simulink model "SerialMaster"  (R2023b)
settings: Solver=FixedStepAuto  StartTime=0.0  StopTime=10.0  FixedStep=1e-3  RelTol=1e-3  EnableMultiTasking=on
undefined symbols (not defined in the file or in its folder): D0, D1, D10, D11, D12, D13, D2, D3, D4, D5, D6, D7, D8, D9, PTA0, PTA1, PTA2, PTB23, PTB9, PTC16, PTC17, PTC2, PTC3, PTC4, PTD0, PTD1, PTD2, PTD3
libraries: frdmk64flib x20, etargetslib x9, dspstat3 x1
settings Model: ExtModeTrigDuration=5  Creator=Mathew  LastModifiedBy=Mathew
settings DataIOCC: InspectSignalLogs=on
settings OptimizationCC: EnhancedBackFolding=on  PassReuseOutputArgsAs=Individual arguments  ZeroExternalMemoryAtStartup=off  ZeroInternalMemoryAtStartup=off  MaxStackSize=64  OptimizeBlockOrder=speed  DifferentSizesBufferReuse=on  OptimizationCustomize=off  EfficientTunableParamExpr=on
settings DebuggingCC: ParameterTunabilityLossMsg=error
settings HardwareCC: ProdBitPerPointer=32  ProdBitPerSizeT=32  ProdBitPerPtrDiffT=32  ProdLargestAtomicInteger=Long  ProdLargestAtomicFloat=Double  ProdWordSize=32  ProdHWDeviceType=ARM Compatible->ARM Cortex
settings SFSimCC: MATLABDynamicMemAlloc=off
settings RTWCC: Description=Embedded Coder  SystemTargetFile=ert.tlc  HardwareBoard=NXP FRDM-K64F  TLCOptions="-aInlineSetEventsForThisBaseRateFcn=TLC_FALSE -aSuppressMultiTaskScheduler=TLC_FALSE  -aRateBasedStepFcn=0"  TemplateMakefile=ert_default_tmf  Toolchain=GNU Tools for ARM Embedded Processors
settings CodeAppCC: ForceParamTrailComments=on  IgnoreCustomStorageClasses=off  OperatorAnnotations=on  SimulinkDataObjDesc=on  SFDataObjDesc=on  InsertBlockDesc=on
settings ERTTargetCC: ExtModeTransport=4  ExtModeMexFile=sendToCommService

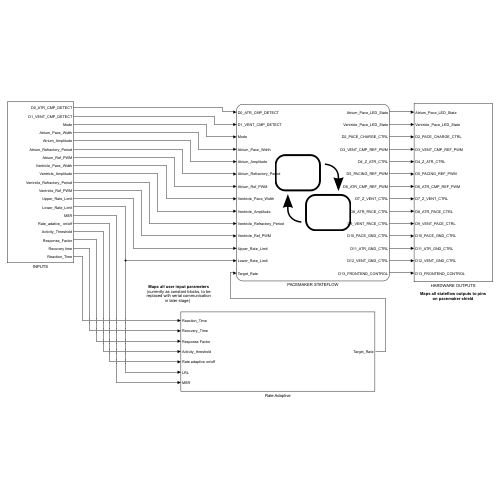
[thumbnail: Simulink's stored preview of the top-level diagram]
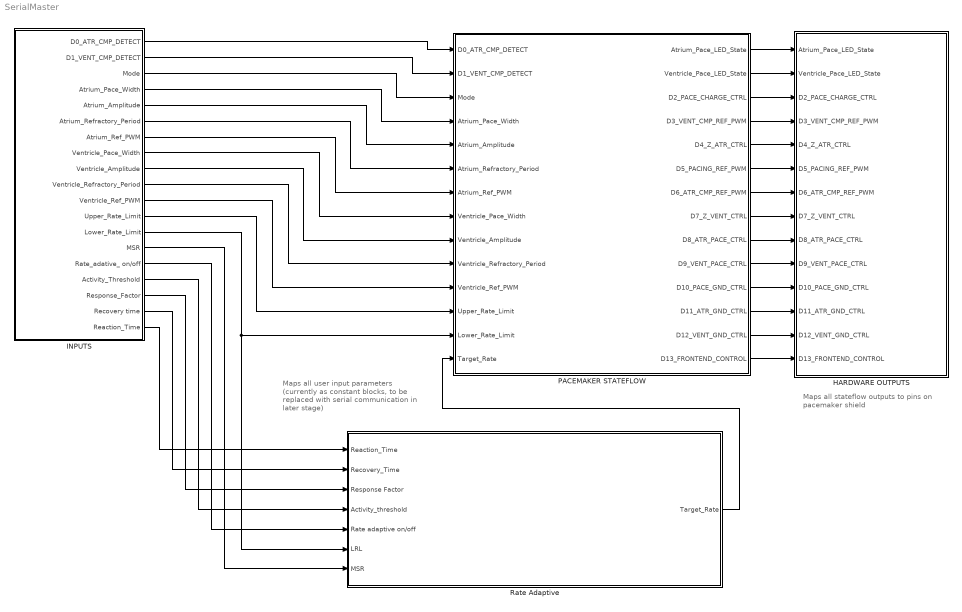
== system SerialMaster ==
  note: Maps all stateflow outputs to pins on pacemaker shield
  note: Maps all user input parameters (currently as constant blocks, to be replaced with serial communication in later stage)
  HARDWARE OUTPUTS : Subsystem
  INPUTS : Subsystem
  PACEMAKER STATEFLOW : Stateflow chart  TreatAsAtomicUnit=on
  Rate Adaptive : Subsystem
  wires:
  Rate Adaptive/1(Target_Rate) -> PACEMAKER STATEFLOW/14(Target_Rate)
  PACEMAKER STATEFLOW/7(D6_ATR_CMP_REF_PWM) -> HARDWARE OUTPUTS/7(D6_ATR_CMP_REF_PWM)
  PACEMAKER STATEFLOW/10(D9_VENT_PACE_CTRL) -> HARDWARE OUTPUTS/10(D9_VENT_PACE_CTRL)
  INPUTS/19(Reaction_Time) -> Rate Adaptive/1(Reaction_Time)
  PACEMAKER STATEFLOW/6(D5_PACING_REF_PWM) -> HARDWARE OUTPUTS/6(D5_PACING_REF_PWM)
  INPUTS/16(Activity_Threshold) -> Rate Adaptive/4(Activity_threshold)
  INPUTS/18(Recovery time) -> Rate Adaptive/2(Recovery_Time)
  INPUTS/15(Rate_adative_ on/off) -> Rate Adaptive/5(Rate adaptive on/off)
  INPUTS/11(Ventricle_Ref_PWM) -> PACEMAKER STATEFLOW/11(Ventricle_Ref_PWM)
  INPUTS/17(Response_Factor) -> Rate Adaptive/3(Response Factor)
  INPUTS/14(MSR) -> Rate Adaptive/7(MSR)
  PACEMAKER STATEFLOW/12(D11_ATR_GND_CTRL) -> HARDWARE OUTPUTS/12(D11_ATR_GND_CTRL)
  INPUTS/13(Lower_Rate_Limit) -> Rate Adaptive/6(LRL), PACEMAKER STATEFLOW/13(Lower_Rate_Limit)
  INPUTS/6(Atrium_Refractory_Period) -> PACEMAKER STATEFLOW/6(Atrium_Refractory_Period)
  PACEMAKER STATEFLOW/4(D3_VENT_CMP_REF_PWM) -> HARDWARE OUTPUTS/4(D3_VENT_CMP_REF_PWM)
  INPUTS/9(Ventricle_Amplitude) -> PACEMAKER STATEFLOW/9(Ventricle_Amplitude)
  INPUTS/10(Ventricle_Refractory_Period) -> PACEMAKER STATEFLOW/10(Ventricle_Refractory_Period)
  PACEMAKER STATEFLOW/14(D13_FRONTEND_CONTROL) -> HARDWARE OUTPUTS/14(D13_FRONTEND_CONTROL)
  INPUTS/7(Atrium_Ref_PWM) -> PACEMAKER STATEFLOW/7(Atrium_Ref_PWM)
  INPUTS/4(Atrium_Pace_Width) -> PACEMAKER STATEFLOW/4(Atrium_Pace_Width)
  INPUTS/3(Mode) -> PACEMAKER STATEFLOW/3(Mode)
  INPUTS/5(Atrium_Amplitude) -> PACEMAKER STATEFLOW/5(Atrium_Amplitude)
  INPUTS/8(Ventricle_Pace_Width) -> PACEMAKER STATEFLOW/8(Ventricle_Pace_Width)
  PACEMAKER STATEFLOW/11(D10_PACE_GND_CTRL) -> HARDWARE OUTPUTS/11(D10_PACE_GND_CTRL)
  PACEMAKER STATEFLOW/8(D7_Z_VENT_CTRL) -> HARDWARE OUTPUTS/8(D7_Z_VENT_CTRL)
  PACEMAKER STATEFLOW/9(D8_ATR_PACE_CTRL) -> HARDWARE OUTPUTS/9(D8_ATR_PACE_CTRL)
  PACEMAKER STATEFLOW/5(D4_Z_ATR_CTRL) -> HARDWARE OUTPUTS/5(D4_Z_ATR_CTRL)
  INPUTS/12(Upper_Rate_Limit) -> PACEMAKER STATEFLOW/12(Upper_Rate_Limit)
  PACEMAKER STATEFLOW/13(D12_VENT_GND_CTRL) -> HARDWARE OUTPUTS/13(D12_VENT_GND_CTRL)
  PACEMAKER STATEFLOW/2(Ventricle_Pace_LED_State) -> HARDWARE OUTPUTS/2(Ventricle_Pace_LED_State)
  INPUTS/2(D1_VENT_CMP_DETECT) -> PACEMAKER STATEFLOW/2(D1_VENT_CMP_DETECT)
  PACEMAKER STATEFLOW/3(D2_PACE_CHARGE_CTRL) -> HARDWARE OUTPUTS/3(D2_PACE_CHARGE_CTRL)
  PACEMAKER STATEFLOW/1(Atrium_Pace_LED_State) -> HARDWARE OUTPUTS/1(Atrium_Pace_LED_State)
  INPUTS/1(D0_ATR_CMP_DETECT) -> PACEMAKER STATEFLOW/1(D0_ATR_CMP_DETECT)

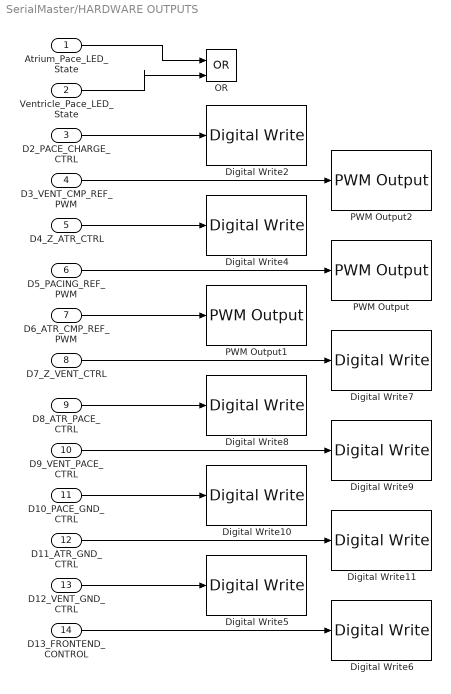
== system SerialMaster/HARDWARE OUTPUTS ==
  Atrium_Pace_LED_State : Inport
  Ventricle_Pace_LED_State : Inport  Port=2
  D2_PACE_CHARGE_CTRL : Inport  Port=3
  D3_VENT_CMP_REF_PWM : Inport  Port=4
  D4_Z_ATR_CTRL : Inport  Port=5
  D5_PACING_REF_PWM : Inport  Port=6
  D6_ATR_CMP_REF_PWM : Inport  Port=7
  D7_Z_VENT_CTRL : Inport  Port=8
  D8_ATR_PACE_CTRL : Inport  Port=9
  D9_VENT_PACE_CTRL : Inport  Port=10
  D10_PACE_GND_CTRL : Inport  Port=11
  D11_ATR_GND_CTRL : Inport  Port=12
  D12_VENT_GND_CTRL : Inport  Port=13
  D13_FRONTEND_CONTROL : Inport  Port=14
  Digital Write10 : frdmk64flib/Digital Write  Whichpin=PTD0 (D10)
  Digital Write11 : frdmk64flib/Digital Write  Whichpin=PTD2 (D11)
  Digital Write2 : frdmk64flib/Digital Write  Whichpin=PTB9 (D2)
  Digital Write4 : frdmk64flib/Digital Write  Whichpin=PTB23 (D4)
  Digital Write5 : frdmk64flib/Digital Write  Whichpin=PTD3 (D12)
  Digital Write6 : frdmk64flib/Digital Write  Whichpin=PTD1 (D13)
  Digital Write7 : frdmk64flib/Digital Write  Whichpin=PTC3 (D7)
  Digital Write8 : frdmk64flib/Digital Write  Whichpin=PTA0 (D8)
  Digital Write9 : frdmk64flib/Digital Write  Whichpin=PTC4 (D9)
  OR : Logic  Operator=OR  IconShape=distinctive  AllPortsSameDT=off  OutDataTypeStr=boolean
  PWM Output : frdmk64flib/PWM Output  Whichpin=PTA2 (D5)  InitialFrequency=2000  InitialDutyCycle=0
  PWM Output1 : frdmk64flib/PWM Output  Whichpin=PTC2 (D6)  InitialFrequency=2000  InitialDutyCycle=0
  PWM Output2 : frdmk64flib/PWM Output  Whichpin=PTA1 (D3)  InitialFrequency=2000  InitialDutyCycle=0
  wires:
  D2_PACE_CHARGE_CTRL/1 -> Digital Write2/1
  D3_VENT_CMP_REF_PWM/1 -> PWM Output2/1
  D4_Z_ATR_CTRL/1 -> Digital Write4/1
  D5_PACING_REF_PWM/1 -> PWM Output/1
  D6_ATR_CMP_REF_PWM/1 -> PWM Output1/1
  D7_Z_VENT_CTRL/1 -> Digital Write7/1
  D8_ATR_PACE_CTRL/1 -> Digital Write8/1
  D9_VENT_PACE_CTRL/1 -> Digital Write9/1
  D10_PACE_GND_CTRL/1 -> Digital Write10/1
  D11_ATR_GND_CTRL/1 -> Digital Write11/1
  D12_VENT_GND_CTRL/1 -> Digital Write5/1
  D13_FRONTEND_CONTROL/1 -> Digital Write6/1
  Atrium_Pace_LED_State/1 -> OR/1
  Ventricle_Pace_LED_State/1 -> OR/2

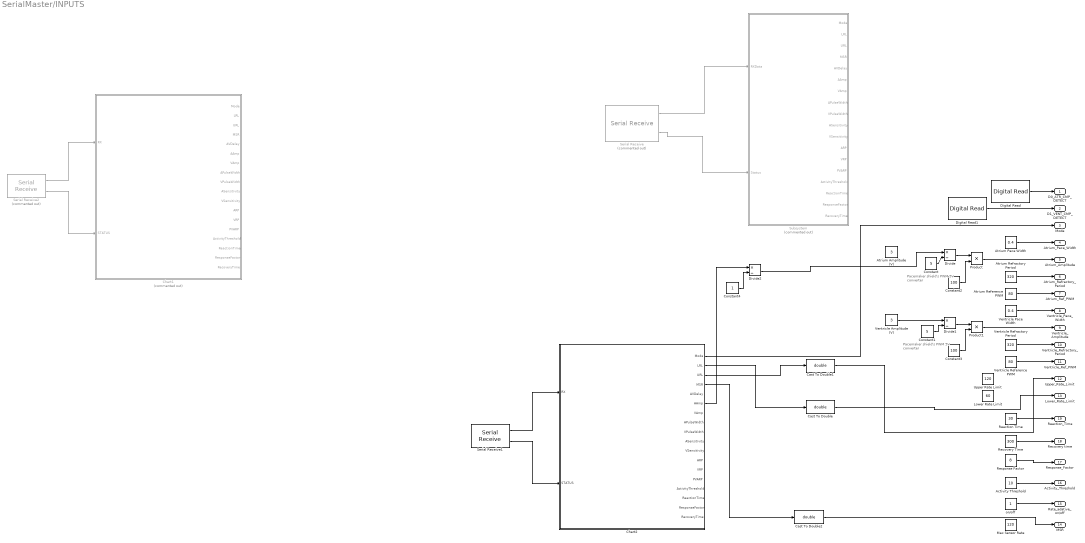
== system SerialMaster/INPUTS ==
  note: Pacemaker shield's PWM 5V converter
  note: Pacemaker shield's PWM 5V converter
  Activity Threshold : Constant  Value=10
  Atrium Amplitude (V) : Constant  Value=3
  Atrium Pace Width : Constant  Value=0.4
  Atrium Reference PWM : Constant  Value=80
  Atrium Refractory Period : Constant  Value=320
  Cast To Double : DataTypeConversion  OutDataTypeStr=double  SaturateOnIntegerOverflow=off  RndMeth=Floor
  Cast To Double1 : DataTypeConversion  OutDataTypeStr=double  SaturateOnIntegerOverflow=off  RndMeth=Floor
  Cast To Double2 : DataTypeConversion  OutDataTypeStr=double  SaturateOnIntegerOverflow=off  RndMeth=Floor
  Chart1 : Stateflow chart  Commented=on  TreatAsAtomicUnit=on
  Chart2 : Stateflow chart  TreatAsAtomicUnit=on
  Constant : Constant  Value=5
  Constant1 : Constant  Value=5
  Constant2 : Constant  Value=100
  Constant3 : Constant  Value=100
  Constant4 : Constant
  Digital Read : frdmk64flib/Digital Read  Whichpin=PTC16 (D0)  SampleTime=-1
  Digital Read1 : frdmk64flib/Digital Read  Whichpin=PTC17 (D1)  SampleTime=-1
  Divide : Product  Inputs=*/
  Divide1 : Product  Inputs=*/
  Divide2 : Product  Inputs=*/
  Lower Rate Limit : Constant  Value=60
  Max Sensor Rate : Constant  Value=120
  Product : Product
  Product1 : Product
  Reaction Time : Constant  Value=30
  Recovery Time : Constant  Value=300
  Response Factor : Constant  Value=8
  Serial Receive : frdmk64flib/Serial Receive  Commented=on  SCIModule=0  Baudrate=uint32(9600)  Parity=None  StopBits=1  HardwareFlowControl=None  ByteOrder=LittleEndian  DataType=uint8  DataLength=3  BlockingMode=off  OutputStatus=on  SampleTime=-1
  Serial Receive1 : frdmk64flib/Serial Receive  SCIModule=0  Baudrate=uint32(9600)  Parity=None  StopBits=1  HardwareFlowControl=None  ByteOrder=LittleEndian  DataType=uint8  DataLength=6  BlockingMode=off  OutputStatus=on  SampleTime=-1
  Serial Receive2 : frdmk64flib/Serial Receive  Commented=on  SCIModule=0  Baudrate=uint32(9600)  Parity=None  StopBits=1  HardwareFlowControl=None  ByteOrder=LittleEndian  DataType=uint8  DataLength=6  BlockingMode=off  OutputStatus=on  SampleTime=-1
  Subsystem : Subsystem  Commented=on
  Upper Rate Limit : Constant  Value=120
  Ventricle Amplitude (V) : Constant  Value=3
  Ventricle Pace Width : Constant  Value=0.4
  Ventricle Reference PWM : Constant  Value=80
  Ventricle Refractory Period : Constant  Value=320
  on/off : Constant
  D0_ATR_CMP_DETECT : Outport
  D1_VENT_CMP_DETECT : Outport  Port=2
  Mode : Outport  Port=3
  Atrium_Pace_Width : Outport  Port=4
  Atrium_Amplitude : Outport  Port=5
  Atrium_Refractory_Period : Outport  Port=6
  Atrium_Ref_PWM : Outport  Port=7
  Ventricle_Pace_Width : Outport  Port=8
  Ventricle_Amplitude : Outport  Port=9
  Ventricle_Refractory_Period : Outport  Port=10
  Ventricle_Ref_PWM : Outport  Port=11
  Upper_Rate_Limit : Outport  Port=12
  Lower_Rate_Limit : Outport  Port=13
  MSR : Outport  Port=14
  Rate_adative_ on/off : Outport  Port=15
  Activity_Threshold : Outport  Port=16
  Response_Factor : Outport  Port=17
  Recovery time : Outport  Port=18
  Reaction_Time : Outport  Port=19
  wires:
  Digital Read/1 -> D0_ATR_CMP_DETECT/1
  Digital Read1/1 -> D1_VENT_CMP_DETECT/1
  Atrium Pace Width/1 -> Atrium_Pace_Width/1
  Atrium Refractory Period/1 -> Atrium_Refractory_Period/1
  Atrium Reference PWM/1 -> Atrium_Ref_PWM/1
  Ventricle Pace Width/1 -> Ventricle_Pace_Width/1
  Ventricle Refractory Period/1 -> Ventricle_Refractory_Period/1
  Ventricle Reference PWM/1 -> Ventricle_Ref_PWM/1
  Constant/1 -> Divide/2
  Ventricle Amplitude (V)/1 -> Divide1/1
  Constant1/1 -> Divide1/2
  Divide/1 -> Product/1
  Product/1 -> Atrium_Amplitude/1
  Constant2/1 -> Product/2
  Divide1/1 -> Product1/1
  Product1/1 -> Ventricle_Amplitude/1
  Constant3/1 -> Product1/2
  Reaction Time/1 -> Reaction_Time/1
  Recovery Time/1 -> Recovery time/1
  Response Factor/1 -> Response_Factor/1
  Activity Threshold/1 -> Activity_Threshold/1
  on/off/1 -> Rate_adative_ on/off/1
  Serial Receive/1 -> Subsystem/1(RXData)
  Serial Receive/2 -> Subsystem/2(Status)
  Cast To Double/1 -> Lower_Rate_Limit/1
  Cast To Double1/1 -> Upper_Rate_Limit/1
  Cast To Double2/1 -> MSR/1
  Chart2/1(Mode) -> Mode/1
  Chart2/2(LRL) -> Cast To Double/1
  Chart2/3(URL) -> Cast To Double1/1
  Chart2/4(MSR) -> Cast To Double2/1
  Serial Receive2/2 -> Chart1/2(STATUS)
  Serial Receive2/1 -> Chart1/1(RX)
  Chart2/6(AAmp) -> Divide2/1
  Divide2/1 -> Divide/1
  Constant4/1 -> Divide2/2
  Serial Receive1/2 -> Chart2/2(STATUS)
  Serial Receive1/1 -> Chart2/1(RX)

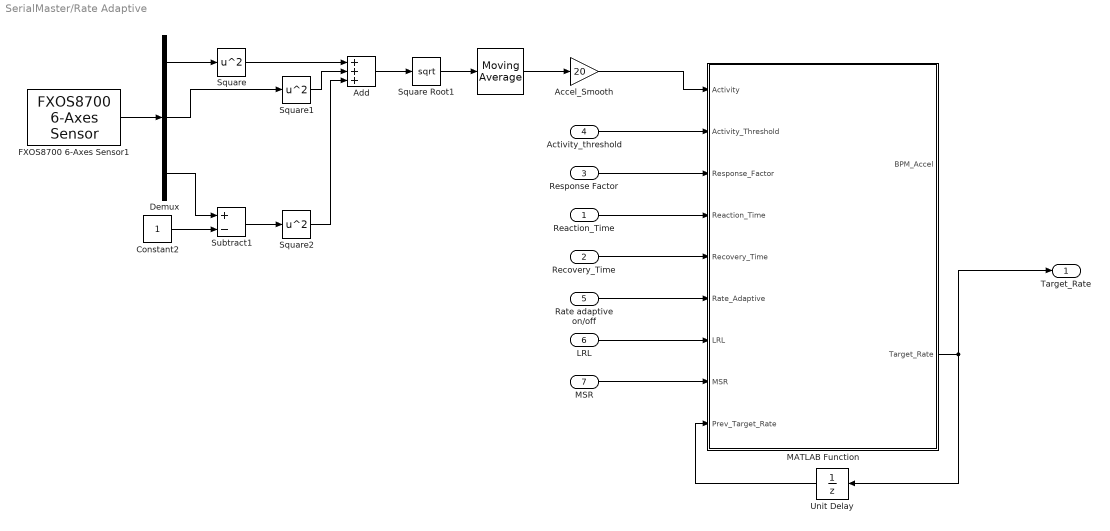
== system SerialMaster/Rate Adaptive ==
  Reaction_Time : Inport
  Recovery_Time : Inport  Port=2
  Response Factor : Inport  Port=3
  Activity_threshold : Inport  Port=4
  Rate adaptive on/off : Inport  Port=5
  LRL : Inport  Port=6
  MSR : Inport  Port=7
  " " : dspstat3/Moving Average  Method=Sliding window  ForgettingFactorPort=off  SpecifyWindowLength=on  WindowLength=300  OverlapLength=299  AllowArbitraryInputLength=off  ForgettingFactor=0.9  SimulateUsing=Code generation
  Accel_Smooth : Gain  Gain=20
  Add : Sum  Inputs=+++
  Constant2 : Constant
  Demux : Demux  Outputs=3
  FXOS8700 6-Axes Sensor1 : frdmk64flib/FXOS8700 6-Axes Sensor  Activesensor=Accelerometer only  ODR=800Hz  HybridODR=400Hz  Accelfullrange=-4g to +4g  SampleTime=-1
  MATLAB Function : MATLAB Function  TreatAsAtomicUnit=on
  Square : Math  Operator=square
  Square Root1 : Sqrt
  Square1 : Math  Operator=square
  Square2 : Math  Operator=square
  Subtract1 : Sum  Inputs=+-
  Unit Delay : UnitDelay  SampleTime=-1  HasFrameUpgradeWarning=on
  Target_Rate : Outport
  wires:
  Rate adaptive on/off/1 -> MATLAB Function/6(Rate_Adaptive)
  FXOS8700 6-Axes Sensor1/1 -> Demux/1
  Demux/1 -> Square/1
  Square1/1 -> Add/2
  Square/1 -> Add/1
  Demux/2 -> Square1/1
  Demux/3 -> Subtract1/1
  Constant2/1 -> Subtract1/2
  Subtract1/1 -> Square2/1
  Square2/1 -> Add/3
  Add/1 -> Square Root1/1
  Square Root1/1 -> " "/1
  " "/1 -> Accel_Smooth/1
  Accel_Smooth/1 -> MATLAB Function/1(Activity)
  Activity_threshold/1 -> MATLAB Function/2(Activity_Threshold)
  Recovery_Time/1 -> MATLAB Function/5(Recovery_Time)
  Response Factor/1 -> MATLAB Function/3(Response_Factor)
  LRL/1 -> MATLAB Function/7(LRL)
  Reaction_Time/1 -> MATLAB Function/4(Reaction_Time)
  MSR/1 -> MATLAB Function/8(MSR)
  MATLAB Function/2(Target_Rate) -> Unit Delay/1, Target_Rate/1
  Unit Delay/1 -> MATLAB Function/9(Prev_Target_Rate)

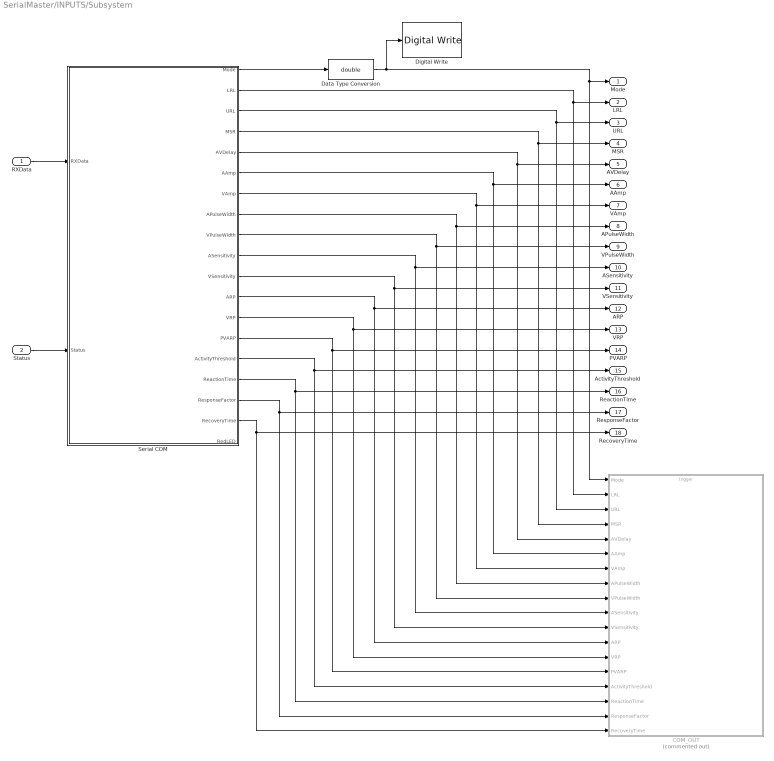
== system SerialMaster/INPUTS/Subsystem ==
  RXData : Inport
  Status : Inport  Port=2
  "COM_OUT " : Subsystem  Commented=on  TreatAsAtomicUnit=on
  Data Type Conversion : DataTypeConversion  OutDataTypeStr=double  SaturateOnIntegerOverflow=off  RndMeth=Floor
  Digital Write : frdmk64flib/Digital Write  Whichpin=RED_LED
  Serial COM : Stateflow chart  TreatAsAtomicUnit=on
      settings: PortSchema="{\"entries\":[{\"content\":{\"sides\":[{\"content\":{\"connectorIds\":[\"In2\",\"In1\"]},\"type\":\"ConnectorPlacement.EquallySpacedRectSide\",\"uuid\":\"c5dd5f70-2f51-479e-a542-05c98a4e4123\"},{\"content\":{\"connectorIds\":[\"Out1\",\"Out2\",\"Out3\",\"Out4\",\"Out5\",\"Out6\",\"Out7\",\"Out8\",\"Out9\",\"Out10\",\"Out11\",\"Out12\",\"Out13\",\"Out14\",\"Out15\",\"Out16\",\"Out17\",\"Out18\",\"Out19\"],\"side\":\"RIGHT\"},\"type\":\"ConnectorPlacement.EquallySpacedRectSide\",\"uuid\":\"909609f0-119b-4759-a7aa-0818fe53bec9\"},{\"content\":{\"side\":\"TOP\"},\"type\":\"ConnectorPlacement.EquallySpacedRectSide\",\"uuid\":\"33a531a6-afe2-48a1-8dbf-b88e90220707\"}]},\"type\":\"ConnectorPlacement.EquallySpacedConnector\",\"uuid\":\"a86a6030-4a17-49da-9f0c-7c45a2a5985f\"}],\"packageUris\":[\"http://schema.mathworks.com/mf0/Connector/R2020b\"],\"version\":\"1.0\"}"
  Mode : Outport  OutDataTypeStr=double
  LRL : Outport  Port=2
  URL : Outport  Port=3
  MSR : Outport  Port=4
  AVDelay : Outport  Port=5
  AAmp : Outport  Port=6
  VAmp : Outport  Port=7
  APulseWidth : Outport  Port=8
  VPulseWidth : Outport  Port=9
  ASensitivity : Outport  Port=10
  VSensitivity : Outport  Port=11
  ARP : Outport  Port=12
  VRP : Outport  Port=13
  PVARP : Outport  Port=14
  ActivityThreshold : Outport  Port=15
  ReactionTime : Outport  Port=16
  ResponseFactor : Outport  Port=17
  RecoveryTime : Outport  Port=18
  wires:
  Status/1 -> Serial COM/1(Status)
  RXData/1 -> Serial COM/2(RXData)
  Serial COM/18(RecoveryTime) -> "COM_OUT "/18(RecoveryTime), RecoveryTime/1
  Serial COM/17(ResponseFactor) -> "COM_OUT "/17(ResponseFactor), ResponseFactor/1
  Serial COM/16(ReactionTime) -> "COM_OUT "/16(ReactionTime), ReactionTime/1
  Serial COM/15(ActivityThreshold) -> "COM_OUT "/15(ActivityThreshold), ActivityThreshold/1
  Serial COM/1(Mode) -> Data Type Conversion/1
  Serial COM/2(LRL) -> "COM_OUT "/2(LRL), LRL/1
  Serial COM/3(URL) -> "COM_OUT "/3(URL), URL/1
  Serial COM/4(MSR) -> "COM_OUT "/4(MSR), MSR/1
  Serial COM/5(AVDelay) -> "COM_OUT "/5(AVDelay), AVDelay/1
  Serial COM/6(AAmp) -> "COM_OUT "/6(AAmp), AAmp/1
  Serial COM/7(VAmp) -> "COM_OUT "/7(VAmp), VAmp/1
  Serial COM/8(APulseWidth) -> "COM_OUT "/8(APulseWidth), APulseWidth/1
  Serial COM/9(VPulseWidth) -> "COM_OUT "/9(VPulseWidth), VPulseWidth/1
  Serial COM/10(ASensitivity) -> "COM_OUT "/10(ASensitivity), ASensitivity/1
  Serial COM/11(VSensitivity) -> "COM_OUT "/11(VSensitivity), VSensitivity/1
  Serial COM/12(ARP) -> "COM_OUT "/12(ARP), ARP/1
  Serial COM/13(VRP) -> "COM_OUT "/13(VRP), VRP/1
  Serial COM/14(PVARP) -> "COM_OUT "/14(PVARP), PVARP/1
  Data Type Conversion/1 -> Digital Write/1, "COM_OUT "/1(Mode), Mode/1

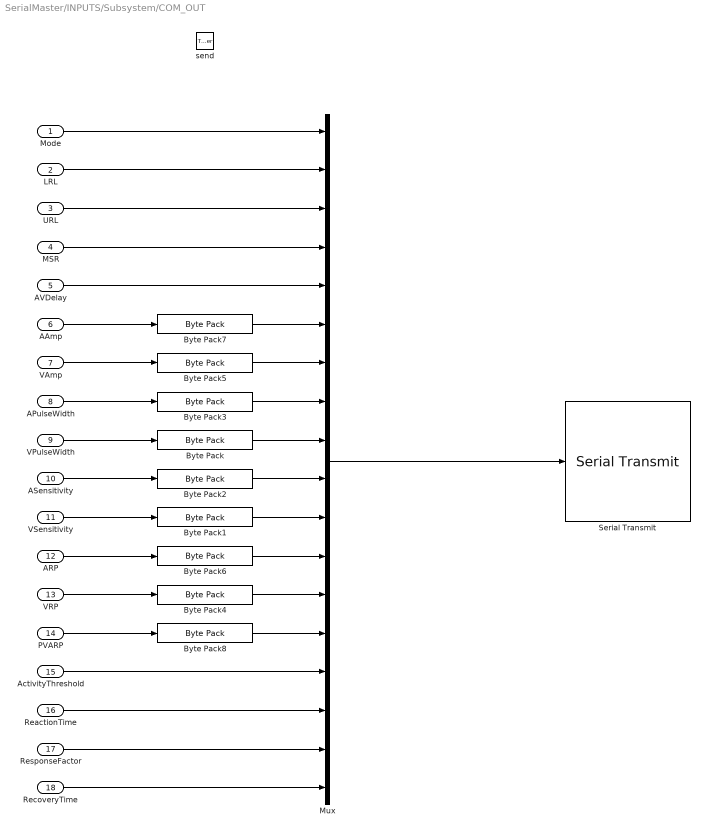
== system SerialMaster/INPUTS/Subsystem/COM_OUT  ==
  Mode : Inport
  LRL : Inport  Port=2
  URL : Inport  Port=3
  MSR : Inport  Port=4
  AVDelay : Inport  Port=5
  AAmp : Inport  Port=6
  VAmp : Inport  Port=7
  APulseWidth : Inport  Port=8
  VPulseWidth : Inport  Port=9
  ASensitivity : Inport  Port=10
  VSensitivity : Inport  Port=11
  ARP : Inport  Port=12
  VRP : Inport  Port=13
  PVARP : Inport  Port=14
  ActivityThreshold : Inport  Port=15
  ReactionTime : Inport  Port=16
  ResponseFactor : Inport  Port=17
  RecoveryTime : Inport  Port=18
  send : TriggerPort  TriggerType=function-call  IsSimulinkFunction=on  FunctionName=send  VariantControl=(inherit)
  Byte Pack{,1..3,5,7} (6 alike) : etargetslib/Byte Pack  datatypes={'single'}  byteAlign=1
  Byte Pack4 : etargetslib/Byte Pack  datatypes={'uint16'}  byteAlign=1
  Byte Pack6 : etargetslib/Byte Pack  datatypes={'uint16'}  byteAlign=1
  Byte Pack8 : etargetslib/Byte Pack  datatypes={'uint16'}  byteAlign=1
  Mux : Mux  Inputs=18
  Serial Transmit : frdmk64flib/Serial Transmit  SCIModule=0  Baudrate=uint32(9600)  Parity=None  StopBits=1  HardwareFlowControl=None  ByteOrder=LittleEndian  BlockingMode=on  OutputStatus=off
  wires:
  VPulseWidth/1 -> Byte Pack/1
  VSensitivity/1 -> Byte Pack1/1
  ASensitivity/1 -> Byte Pack2/1
  APulseWidth/1 -> Byte Pack3/1
  VRP/1 -> Byte Pack4/1
  VAmp/1 -> Byte Pack5/1
  ARP/1 -> Byte Pack6/1
  AAmp/1 -> Byte Pack7/1
  PVARP/1 -> Byte Pack8/1
  Mux/1 -> Serial Transmit/1
  Byte Pack8/1 -> Mux/14
  Byte Pack4/1 -> Mux/13
  Byte Pack6/1 -> Mux/12
  Byte Pack1/1 -> Mux/11
  Byte Pack2/1 -> Mux/10
  Byte Pack/1 -> Mux/9
  Byte Pack3/1 -> Mux/8
  Byte Pack5/1 -> Mux/7
  Byte Pack7/1 -> Mux/6
  AVDelay/1 -> Mux/5
  MSR/1 -> Mux/4
  URL/1 -> Mux/3
  LRL/1 -> Mux/2
  Mode/1 -> Mux/1
  ActivityThreshold/1 -> Mux/15
  ReactionTime/1 -> Mux/16
  ResponseFactor/1 -> Mux/17
  RecoveryTime/1 -> Mux/18

== stateflow chart SerialMaster/INPUTS/Subsystem/Serial COM ==
  state Preset
    entry:
    Mode=1;   %int unit8
    LRL=60;   %BPM uint8
    URL=120;   %BPM uint8
    MSR=120;   %BPM uint8
    AVDelay=150;   %ms uint8
    AAmp=3.5;   %V single
    VAmp=3.5;   %V single
    APulseWidth=0.4;   %ms single
    VPulseWidth=0.4;   %ms single
    ASensitivity=0.75;   %mV single
    VSensitivity=2.5;   %mV single
    ARP=250;   %ms uint16
    VRP=320;   %ms uint16
    PVARP=320;   %ms uint16
    ActivityThreshold=4;   %int uint8
    ReactionTime=30;   %s uint8
    ResponseFactor=8   %int uint8
    RecoveryTime=5;   %min uint8
  state SaveData
    entry:
    Mode=RXData(3);   %int unit8
    %LRL=LRLIN;   %BPM uint8
    %URL=URLIN;   %BPM uint8
    %MSR=MSRIN;   %BPM uint8
    %AVDelay=AVDELAYIN;   %ms uint8
    %AAmp=AAMPIN;   %V single
    %VAmp=VAMPIN;   %V single
    %APulseWidth= APWIN;   %ms single
    %VPulseWidth= VPWIN;   %ms single
    %ASensitivity= ASIN;   %mV single
    %VSensitivity= VSIN;   %mV single
    %ARP= ARPIN;   %ms uint16
    %VRP= VRPIN;   %ms uint16
    %PVARP=PVARPIN;   %ms uint16
    %ActivityThreshold=ACTTHRESHIN;   %int uint8
    %ReactionTime=REACTIN;   %s uint8
    %ResponseFactor=RESPONSEIN   %int uint8
    %RecoveryTime=RECOVERYIN;   %min uint8
  state Standby
  state CheckSync
    entry:
  state CheckFunction
    entry:
    RedLED=true;
  state ReturnData [commented out]
    entry:
    send()
  (default) -> Preset
  CheckFunction -> SaveData : [RXData(2)==27]
  Standby -> CheckSync
  Preset -> Standby
  CheckSync -> CheckFunction : [RXData(1)==59]
  SaveData -> Standby
  ReturnData -> Standby [commented out]
  CheckFunction -> ReturnData [commented out] : [FUNCIN==hex2dec('22')]
  data: Mode output uint8; LRL output uint8; URL output uint8; MSR output uint8; AVDelay output uint8; AAmp output single; VAmp output single; APulseWidth output single; VPulseWidth output single; ASensitivity output single; VSensitivity output single; ARP output uint16; VRP output uint16; PVARP output uint16; Status input size=1; RXData input; ActivityThreshold output uint8; ReactionTime output uint8; ResponseFactor output uint8; RecoveryTime output uint8; RedLED output

== matlab function SerialMaster/Rate Adaptive/MATLAB Function ==
  data: Activity input; Activity_Threshold input; BPM_Accel output; Response_Factor input; Reaction_Time input; Recovery_Time input; Rate_Adaptive input; LRL input; MSR input; Prev_Target_Rate input; Target_Rate output
function [BPM_Accel,Target_Rate]  = Rate_Response(Activity,Activity_Threshold,Response_Factor,Reaction_Time,Recovery_Time,Rate_Adaptive,LRL,MSR,Prev_Target_Rate)

Activity_Factor = 10*Response_Factor*(Activity-Activity_Threshold); %negative if below threshold

derivative_Activity=diff(Activity);

if(Rate_Adaptive==0)
    BPM_Accel=0;
elseif(derivative_Activity>=0)              %if increasing
    BPM_Accel=Activity_Factor/Reaction_Time;
else                                        %if decreasing
    BPM_Accel=Activity_Factor/Recovery_Time;
end

Target_Rate=BPM_Accel*(1e-3)+Prev_Target_Rate;

if(Target_Rate<LRL)
    Target_Rate=LRL;
elseif(Target_Rate>MSR)
    Target_Rate=MSR;
end

== stateflow chart SerialMaster/PACEMAKER STATEFLOW ==
  state AOO
    state Pace
      entry:
      D5_PACING_REF_PWM = 0
      D2_PACE_CHARGE_CTRL=0;
      D10_PACE_GND_CTRL=1;
      D8_ATR_PACE_CTRL=1;
      D11_ATR_GND_CTRL=0;
      D4_Z_ATR_CTRL=0;
      D7_Z_VENT_CTRL=0;
      D12_VENT_GND_CTRL=0;
      D9_VENT_PACE_CTRL=0;
      Atrium_Pace_LED_State=1;
    state Refractory
      entry:
      D10_PACE_GND_CTRL=1;
      D9_VENT_PACE_CTRL=0;
      D4_Z_ATR_CTRL=0;
      D7_Z_VENT_CTRL=0;
      D8_ATR_PACE_CTRL=0;
      D11_ATR_GND_CTRL=1;
      D12_VENT_GND_CTRL=0;
      D2_PACE_CHARGE_CTRL=1;
      D5_PACING_REF_PWM = Atrium_Amplitude
      Atrium_Pace_LED_State=0;
      Standby_Period=(1/(Target_Rate))*30000
    (default) -> AOO.Refractory
    AOO.Pace -> AOO.Refractory : [after(Atrium_Pace_Width,msec)]
    AOO.Refractory -> AOO.Pace : [after(Standby_Period,msec)]
  state AAI
    state Pace
      entry:
      D5_PACING_REF_PWM = 0
      D2_PACE_CHARGE_CTRL=0;
      D10_PACE_GND_CTRL=1;
      D8_ATR_PACE_CTRL=1;
      D11_ATR_GND_CTRL=0;
      D4_Z_ATR_CTRL=0;
      D7_Z_VENT_CTRL=0;
      D12_VENT_GND_CTRL=0;
      D9_VENT_PACE_CTRL=0;
      Atrium_Pace_LED_State=1;
    state Refractory
      entry:
      D5_PACING_REF_PWM = Atrium_Amplitude
      D10_PACE_GND_CTRL=1;
      D9_VENT_PACE_CTRL=0;
      D4_Z_ATR_CTRL=0;
      D7_Z_VENT_CTRL=0;
      D8_ATR_PACE_CTRL=0;
      D11_ATR_GND_CTRL=1;
      D12_VENT_GND_CTRL=0;
      D2_PACE_CHARGE_CTRL=1;
      D6_ATR_CMP_REF_PWM = Atrium_Ref_PWM;
      Atrium_Pace_LED_State=0;
      Standby_Period=30000/(Target_Rate)
    state waiting
    state Sense
    AAI.Pace -> AAI.Refractory : [after(Atrium_Pace_Width,msec)]
    (default) -> AAI.Refractory
    AAI.waiting -> AAI.Sense : [[after(Atrium_Refractory_Period,msec)]]
    AAI.Refractory -> AAI.waiting
    AAI.Sense -> AAI.waiting [order 2] : [D0_ATR_CMP_DETECT == 1]
    AAI.Sense -> AAI.Pace [order 1] : after(Standby_Period-Atrium_Pace_Width-Atrium_Refractory_Period,msec)
  state VOO
    state Pace
      entry:
      D5_PACING_REF_PWM = 0
      D2_PACE_CHARGE_CTRL=0;
      D10_PACE_GND_CTRL=1;
      D8_ATR_PACE_CTRL=0;
      D11_ATR_GND_CTRL=0;
      D4_Z_ATR_CTRL=0;
      D7_Z_VENT_CTRL=0;
      D12_VENT_GND_CTRL=0;
      D9_VENT_PACE_CTRL=1;
      Ventricle_Pace_LED_State=1;
    state Refractory
      entry:
      D10_PACE_GND_CTRL=1;
      D9_VENT_PACE_CTRL=0;
      D4_Z_ATR_CTRL=0;
      D7_Z_VENT_CTRL=0;
      D8_ATR_PACE_CTRL=0;
      D11_ATR_GND_CTRL=0;
      D12_VENT_GND_CTRL=1;
      D2_PACE_CHARGE_CTRL=1;
      D5_PACING_REF_PWM = Ventricle_Amplitude
      Ventricle_Pace_LED_State=0;
      Standby_Period=(1/(Lower_Rate_Limit))*30000
    (default) -> VOO.Refractory
    VOO.Pace -> VOO.Refractory : [after(Ventricle_Pace_Width,msec)]
    VOO.Refractory -> VOO.Pace : [after(Standby_Period,msec)]
  state VVI
    state Pace
      entry:
      D5_PACING_REF_PWM = 0
      D2_PACE_CHARGE_CTRL=0;
      D10_PACE_GND_CTRL=1;
      D8_ATR_PACE_CTRL=0;
      D11_ATR_GND_CTRL=0;
      D4_Z_ATR_CTRL=0;
      D7_Z_VENT_CTRL=0;
      D12_VENT_GND_CTRL=0;
      D9_VENT_PACE_CTRL=1;
    state Refractory
      entry:
      D5_PACING_REF_PWM = Ventricle_Amplitude
      D10_PACE_GND_CTRL=1;
      D9_VENT_PACE_CTRL=0;
      D4_Z_ATR_CTRL=0;
      D7_Z_VENT_CTRL=0;
      D8_ATR_PACE_CTRL=0;
      D11_ATR_GND_CTRL=0;
      D12_VENT_GND_CTRL=1;
      D2_PACE_CHARGE_CTRL=1;
      D3_VENT_CMP_REF_PWM = Ventricle_Ref_PWM;
      Ventricle_Pace_LED_State=0;
      Standby_Period=30000/(Target_Rate)
    state Sense
    state waiting
    VVI.Pace -> VVI.Refractory : [after(Ventricle_Pace_Width,msec)]
    (default) -> VVI.Refractory
    VVI.waiting -> VVI.Sense : [[after(Ventricle_Refractory_Period,msec)]]
    VVI.Refractory -> VVI.waiting
    VVI.Sense -> VVI.Pace [order 1] : after(Standby_Period-Ventricle_Pace_Width-Ventricle_Refractory_Period,msec)
    VVI.Sense -> VVI.waiting [order 2] : [D1_VENT_CMP_DETECT == 1]
  (default) -> AOO
  AOO -> AAI [order 1] : [Mode==2]
  AAI -> AOO [order 2] : [Mode==0]
  AOO -> VVI [order 3] : [Mode==3]
  VOO -> AAI [order 3] : [Mode==2]
  VOO -> AOO [order 1] : [Mode==0]
  AOO -> VOO [order 2] : [Mode==1]
  VVI -> AOO [order 3] : [Mode==0]
  AAI -> VOO [order 3] : [Mode==1]
  VVI -> AAI [order 2] : [Mode==2]
  AAI -> VVI [order 1] : [Mode==3]
  VOO -> VVI [order 2] : [Mode==3]
  VVI -> VOO [order 1] : [Mode==1]
  data: D0_ATR_CMP_DETECT input; D1_VENT_CMP_DETECT input; Mode input; Atrium_Pace_Width input; Atrium_Amplitude input; Atrium_Refractory_Period input; Atrium_Ref_PWM input; Ventricle_Pace_Width input; Ventricle_Amplitude input; Ventricle_Refractory_Period input; Ventricle_Ref_PWM input; Atrium_Pace_LED_State output; Ventricle_Pace_LED_State output; D2_PACE_CHARGE_CTRL output; D3_VENT_CMP_REF_PWM output; D4_Z_ATR_CTRL output; D5_PACING_REF_PWM output; D6_ATR_CMP_REF_PWM output; D7_Z_VENT_CTRL output; D8_ATR_PACE_CTRL output; D9_VENT_PACE_CTRL output; D10_PACE_GND_CTRL output; D11_ATR_GND_CTRL output; D12_VENT_GND_CTRL output; Upper_Rate_Limit input; Lower_Rate_Limit input; Standby_Period local; D13_FRONTEND_CONTROL output boolean =true; Target_Rate input

== stateflow chart SerialMaster/INPUTS/Chart2 ==
  state Default
    entry:
    Mode=0;   %int unit8
    LRL=60;   %BPM uint8
    URL=120;   %BPM uint8
    MSR=120;   %BPM uint8
    AVDelay=150;   %ms uint8
    AAmp=3.5;   %V single
    VAmp=3.5;   %V single
    APulseWidth=0.4;   %ms single
    VPulseWidth=0.4;   %ms single
    ASensitivity=0.75;   %mV single
    VSensitivity=2.5;   %mV single
    ARP=250;   %ms uint16
    VRP=320;   %ms uint16
    PVARP=320;   %ms uint16
    ActivityThreshold=4;   %int uint8
    ReactionTime=30;   %s uint8
    ResponseFactor=8   %int uint8
    RecoveryTime=5;   %min uint8
  state entry_1
    exit:
    SYNC=RX(1);
    FUNC=RX(2);
    MODE=RX(3);
    LRLIN=RX(4);
    URLIN=RX(5);
    MSRIN=RX(6);
  state name
  state hehe
  state entry_
    Mode=MODE;
    LRL=LRLIN;
    URL=URLIN;
    MSR=MSRIN;
  (default) -> Default
  Default -> entry_1
  entry_1 -> name : [STATUS==0]
  hehe -> entry_ : [FUNC==45]
  name -> hehe : [SYNC==59]
  entry_ -> entry_1
  data: RX input; Mode output; FUNC local; SYNC local; MODE local; STATUS input; LRL output; URL output; MSR output; AVDelay output; AAmp output; VAmp output; APulseWidth output; VPulseWidth output; ASensitivity output; VSensitivity output; ARP output; VRP output; PVARP output; LRLIN local; ActivityThreshold output; ReactionTime output; ResponseFactor output; RecoveryTime output; MSRIN local; URLIN local; AAMP local size=1; AVDELAY local; test local

== stateflow chart SerialMaster/INPUTS/Chart1 ==
  state Default
    entry:
    Mode=0;   %int unit8
    LRL=60;   %BPM uint8
    URL=120;   %BPM uint8
    MSR=120;   %BPM uint8
    AVDelay=150;   %ms uint8
    AAmp=3.5;   %V single
    VAmp=3.5;   %V single
    APulseWidth=0.4;   %ms single
    VPulseWidth=0.4;   %ms single
    ASensitivity=0.75;   %mV single
    VSensitivity=2.5;   %mV single
    ARP=250;   %ms uint16
    VRP=320;   %ms uint16
    PVARP=320;   %ms uint16
    ActivityThreshold=4;   %int uint8
    ReactionTime=30;   %s uint8
    ResponseFactor=8   %int uint8
    RecoveryTime=5;   %min uint8
  state entry_1
    exit:
    SYNC=RX(1);
    FUNC=RX(2);
    MODE=RX(3);
    LRLIN=RX(4);
    URLIN=RX(5);
    MSRIN=RX(6);
  state name
  state hehe
  state entry_
    Mode=MODE;
    LRL=LRLIN;
    URL=URLIN;
    MSR=MSRIN;
  (default) -> Default
  Default -> entry_1
  entry_1 -> name : [STATUS==0]
  hehe -> entry_ : [FUNC==45]
  name -> hehe : [SYNC==59]
  entry_ -> entry_1
  data: RX input; Mode output; FUNC local; SYNC local; MODE local; STATUS input; LRL output; URL output; MSR output; AVDelay output; AAmp output; VAmp output; APulseWidth output; VPulseWidth output; ASensitivity output; VSensitivity output; ARP output; VRP output; PVARP output; LRLIN local; ActivityThreshold output; ReactionTime output; ResponseFactor output; RecoveryTime output; MSRIN local; URLIN local; AAMP local size=1; AVDELAY local; test local
